simulink model "Test_Decoder_4_to_16"  (R2023a)
settings: Solver=ode45  StartTime=0.0  StopTime=len  RelTol=1e-3  EnableMultiTasking=on
libraries: simulink x2, Decoders_Lib x1
settings Model: Creator=N  LastModifiedBy=Jozko Mrkvicka
settings SolverCC: AlgebraicLoopSolver=TrustRegion
settings DataIOCC: SaveFormat=Array  ReturnWorkspaceOutputs=off
settings OptimizationCC: LifeSpan=inf
settings DebuggingCC: UnconnectedInputMsg=warning  UnconnectedOutputMsg=warning  UnconnectedLineMsg=warning  SFUnexpectedBacktrackingDiag=warning  SFNoUnconditionalDefaultTransitionDiag=warning  SFExecutionAtInitializationDiag=none  ArithmeticOperatorsInVariantConditions=warning
settings HardwareCC: ProdWordSize=32
settings SFSimCC: SimUseLocalCustomCode=off  CustomCodeUndefinedFunction=UseInterfaceOnly
settings RTWCC: RTWUseLocalCustomCode=off
settings CodeAppCC: StateflowObjectComments=on
settings GRTTargetCC: TargetLangStandard=C89/C90 (ANSI)
settings ConfigComp: CovMetricSettings=dw  CovSaveCumulativeToWorkspaceVar=on  CovSaveSingleToWorkspaceVar=on  CovExternalEMLEnable=off

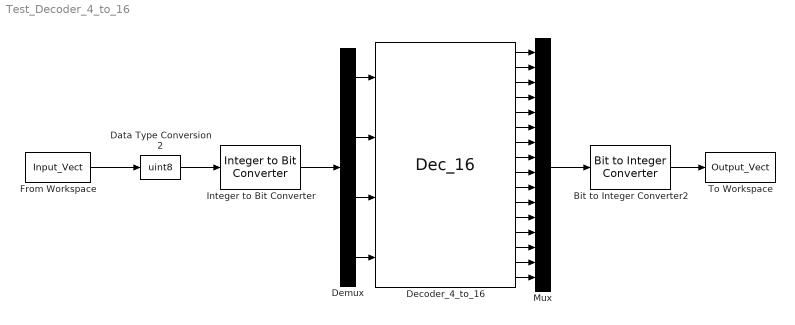
== system Test_Decoder_4_to_16 ==
  Bit to Integer Converter2 : simulink/Logic and Bit Operations/Bit to Integer Converter  nbits=16  bitOrder=MSB first  signedOutputValues=Unsigned  outDtype=uint16  outDtypeSigned=Inherit via internal rule
      settings: LibrarySourceBlock=|
      | commutil2/Bit to Integer
      | Converter
  Data Type Conversion2 : DataTypeConversion  OutDataTypeStr=uint8  SaturateOnIntegerOverflow=off  RndMeth=Floor
  Decoder_4_to_16 : Decoders_Lib/Dec_16  SystemSampleTime=-1  VariantActivationTime=update diagram  Latency=0  AutoFrameSizeCalculation=off
  Demux : Demux
  From Workspace : FromWorkspace  VariableName=Input_Vect  SampleTime=1  Interpolate=off  ZeroCross=off  OutputAfterFinalValue=Holding final value
  Integer to Bit Converter : simulink/Logic and Bit Operations/Integer to Bit Converter  nbits=4  signedInputValues=Unsigned  bitOrder=MSB first  outDtype=uint8
      settings: LibrarySourceBlock=|
      | commutil2/Integer to Bit
      | Converter
  Mux : Mux  Inputs=16
  To Workspace : ToWorkspace  VariableName=Output_Vect  SampleTime=1
  wires:
  Decoder_4_to_16/1 -> Mux/1
  Decoder_4_to_16/2 -> Mux/2
  Decoder_4_to_16/3 -> Mux/3
  Decoder_4_to_16/4 -> Mux/4
  Decoder_4_to_16/5 -> Mux/5
  Decoder_4_to_16/6 -> Mux/6
  Decoder_4_to_16/7 -> Mux/7
  Decoder_4_to_16/8 -> Mux/8
  Decoder_4_to_16/9 -> Mux/9
  Decoder_4_to_16/10 -> Mux/10
  Decoder_4_to_16/11 -> Mux/11
  Decoder_4_to_16/12 -> Mux/12
  Decoder_4_to_16/13 -> Mux/13
  Decoder_4_to_16/14 -> Mux/14
  Decoder_4_to_16/15 -> Mux/15
  Decoder_4_to_16/16 -> Mux/16
  Demux/1 -> Decoder_4_to_16/1
  Demux/2 -> Decoder_4_to_16/2
  Demux/3 -> Decoder_4_to_16/3
  Demux/4 -> Decoder_4_to_16/4
  Integer to Bit Converter/1 -> Demux/1
  Data Type Conversion2/1 -> Integer to Bit Converter/1
  Mux/1 -> Bit to Integer Converter2/1
  From Workspace/1 -> Data Type Conversion2/1
  Bit to Integer Converter2/1 -> To Workspace/1
